simulink model "model5"  (R2022a)
settings: Solver=FixedStepAuto  StartTime=0.0  StopTime=20  FixedStep=1e-4  RelTol=1e-3
PreLoadFcn:
  | m = 3.600;     % kg
  | k = 400;    % N/m
  | b = 10;      % Ns/m
  | x0=1; %m
model workspace (MAT data in the model file):
  b1 = 10
  b2 = 10
  downSpringHeight = 10
  g = 9.81
  groundHeight = 100
  k1 = 400
  k2 = 400
  m1 = 3.6
  m1IniHeight = 10
  m2 = 3.6
  m3 = 3.6
  upSpringHeight = 10
settings Model: Creator=Tsing  LastModifiedBy=Tsing

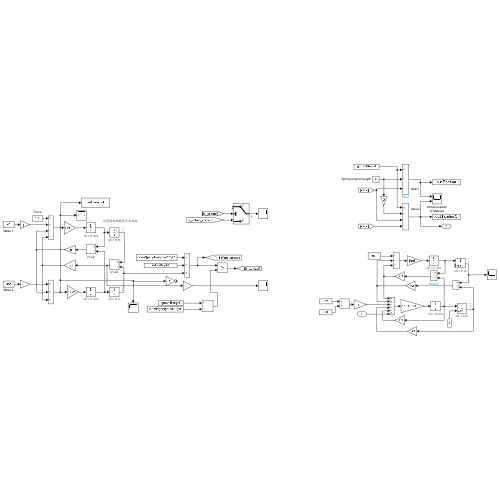
[thumbnail: Simulink's stored preview of the top-level diagram]
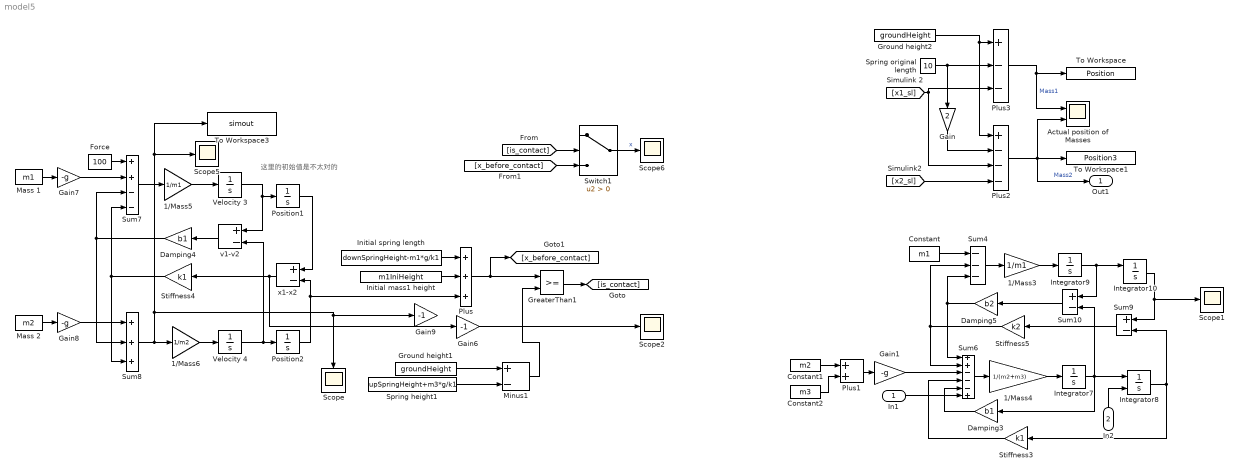
== system model5 ==
  note: 这里的初始值是不太对的
  In1 : Inport
  In2 : Inport  Port=2
  1/Mass3 : Gain  Gain=1/m1  SaturateOnIntegerOverflow=on  OutDataTypeStr=Inherit: Same as input  ParamDataTypeStr=Inherit: Same as input
  1/Mass4 : Gain  Gain=1/(m2+m3)  SaturateOnIntegerOverflow=on  OutDataTypeStr=Inherit: Same as input  ParamDataTypeStr=Inherit: Same as input
  1/Mass5 : Gain  Gain=1/m1  SaturateOnIntegerOverflow=on  OutDataTypeStr=Inherit: Same as input  ParamDataTypeStr=Inherit: Same as input
  1/Mass6 : Gain  Gain=1/m2  SaturateOnIntegerOverflow=on  OutDataTypeStr=Inherit: Same as input  ParamDataTypeStr=Inherit: Same as input
  Actual position of Masses : Scope  NumInputPorts=2
  Constant : Constant  Value=m1
  Constant1 : Constant  Value=m2
  Constant2 : Constant  Value=m3
  Damping3 : Gain  Gain=b1  SaturateOnIntegerOverflow=on  OutDataTypeStr=Inherit: Same as input  ParamDataTypeStr=Inherit: Same as input
  Damping4 : Gain  Gain=b1  SaturateOnIntegerOverflow=on  OutDataTypeStr=Inherit: Same as input  ParamDataTypeStr=Inherit: Same as input
  Damping5 : Gain  Gain=b2  SaturateOnIntegerOverflow=on  OutDataTypeStr=Inherit: Same as input  ParamDataTypeStr=Inherit: Same as input
  Force : Constant  Value=100
  Gain : Gain  Gain=2
  Gain1 : Gain  Gain=-g
  Gain6 : Gain  Gain=-1
  Gain7 : Gain  Gain=-g
  Gain8 : Gain  Gain=-g
  Gain9 : Gain  Gain=-1
  GreaterThan1 : RelationalOperator  OutDataTypeStr=boolean  RndMeth=Simplest  InputSameDT=off
  Ground height1 : Constant  Value=groundHeight
  Ground height2 : Constant  Value=groundHeight
  Initial mass1 height : Constant  Value=m1IniHeight
  Initial spring length : Constant  Value=downSpringHeight-m1*g/k1
  Integrator10 : Integrator  InitialConditionSource=external
      settings: AttributesFormatString=x0 = %<InitialCondition> m
  Integrator7 : Integrator
      settings: AttributesFormatString=v0 = %<InitialCondition> m/s
  Integrator8 : Integrator  InitialConditionSource=external
      settings: AttributesFormatString=x0 = %<InitialCondition> m
  Integrator9 : Integrator
      settings: AttributesFormatString=v0 = %<InitialCondition> m/s
  Mass 1 : Constant  Value=m1
  Mass 2 : Constant  Value=m2
  Minus1 : Sum  Inputs=+-
  Plus : Sum  Inputs=+++
  Plus1 : Sum
  Plus2 : Sum  Inputs=+---
  Plus3 : Sum  Inputs=+--
  Position1 : Integrator
      settings: AttributesFormatString=x0 = %<InitialCondition> m
  Position2 : Integrator
      settings: AttributesFormatString=x0 = %<InitialCondition> m
  Scope{,1..2,5..6} (5 alike) : Scope
  Spring height1 : Constant  Value=upSpringHeight+m3*g/k1
  Spring original length : Constant  Value=10
  Stiffness3 : Gain  Gain=k1  SaturateOnIntegerOverflow=on  OutDataTypeStr=Inherit: Same as input  ParamDataTypeStr=Inherit: Same as input
  Stiffness4 : Gain  Gain=k1  SaturateOnIntegerOverflow=on  OutDataTypeStr=Inherit: Same as input  ParamDataTypeStr=Inherit: Same as input
  Stiffness5 : Gain  Gain=k2  SaturateOnIntegerOverflow=on  OutDataTypeStr=Inherit: Same as input  ParamDataTypeStr=Inherit: Same as input
  Sum10 : Sum  Inputs=+-  InputSameDT=on  SaturateOnIntegerOverflow=on  OutDataTypeStr=Inherit: Same as first input
  Sum4 : Sum  Inputs=---  InputSameDT=on  SaturateOnIntegerOverflow=on  OutDataTypeStr=Inherit: Same as first input
  Sum6 : Sum  Inputs=++---+  InputSameDT=on  SaturateOnIntegerOverflow=on  OutDataTypeStr=Inherit: Same as first input
  Sum7 : Sum  Inputs=++--  InputSameDT=on  SaturateOnIntegerOverflow=on  OutDataTypeStr=Inherit: Same as first input
  Sum8 : Sum  Inputs=+++  InputSameDT=on  SaturateOnIntegerOverflow=on  OutDataTypeStr=Inherit: Same as first input
  Sum9 : Sum  Inputs=+-  InputSameDT=on  SaturateOnIntegerOverflow=on  OutDataTypeStr=Inherit: Same as first input
  Switch1 : Switch  Criteria=u2 > Threshold  SaturateOnIntegerOverflow=off  InputSameDT=off
  To Workspace : ToWorkspace  VariableName=Position  SaveFormat=Timeseries  SampleTime=-1
  To Workspace1 : ToWorkspace  VariableName=Position3  SaveFormat=Timeseries  SampleTime=-1
  To Workspace3 : ToWorkspace  VariableName=simout  SaveFormat=Timeseries  SampleTime=-1
  Velocity 3 : Integrator
      settings: AttributesFormatString=v0 = %<InitialCondition> m/s
  Velocity 4 : Integrator
      settings: AttributesFormatString=v0 = %<InitialCondition> m/s
  v1-v2 : Sum  Inputs=+-
  x1-x2 : Sum  Inputs=+-
  Out1 : Outport
  wires:
  Gain8/1 -> Sum8/1
  Mass 2/1 -> Gain8/1
  Sum8/1 -> To Workspace3/1, Scope5/1, Gain9/1, Scope/1, 1/Mass6/1
  Stiffness4/1 -> Sum7/4, Sum8/3
  Velocity 3/1 -> Position1/1, v1-v2/1
  Damping4/1 -> Sum7/3, Sum8/2
  Force/1 -> Sum7/1
  v1-v2/1 -> Damping4/1
  1/Mass5/1 -> Velocity 3/1
  Sum7/1 -> 1/Mass5/1
  Velocity 4/1 -> Position2/1, v1-v2/2
  Position1/1 -> x1-x2/1
  1/Mass6/1 -> Velocity 4/1
  Mass 1/1 -> Gain7/1
  Gain7/1 -> Sum7/2
  Position2/1 -> Plus/3, x1-x2/2
  x1-x2/1 -> Gain6/1, Stiffness4/1
  Spring height1/1 -> Minus1/2
  Ground height1/1 -> Minus1/1
  Plus/1 -> [x_before_contact], GreaterThan1/1
  Initial spring length/1 -> Plus/1
  Minus1/1 -> GreaterThan1/2
  GreaterThan1/1 -> [is_contact]
  Initial mass1 height/1 -> Plus/2
  Integrator10/1 -> Scope1/1, Sum9/1
  Stiffness3/1 -> Sum6/4
  Plus3/1 -> To Workspace/1, Actual position of Masses/1  "Mass1"
  Ground height2/1 -> Plus2/1, Plus3/1
  [x1_sl] -> Plus2/3, Plus3/3
  Sum9/1 -> Stiffness5/1
  1/Mass4/1 -> Integrator7/1
  In2/1 -> Integrator8/2
  Integrator7/1 -> Sum10/2, Integrator8/1, Damping3/1
  Gain/1 -> Plus2/2
  Spring original length/1 -> Gain/1, Plus3/2
  [x2_sl] -> Plus2/4
  Stiffness5/1 -> Sum6/2, Sum4/2
  Damping3/1 -> Sum6/5
  Integrator9/1 -> Integrator10/1, Sum10/1
  In1/1 -> Sum6/6
  Constant/1 -> Sum4/1
  Integrator8/1 -> Sum9/2, Stiffness3/1
  Plus2/1 -> Out1/1, To Workspace1/1, Actual position of Masses/2  "Mass2"
  Sum6/1 -> 1/Mass4/1
  Damping5/1 -> Sum4/3, Sum6/1
  Sum10/1 -> Damping5/1
  1/Mass3/1 -> Integrator9/1
  Sum4/1 -> 1/Mass3/1
  [is_contact] -> Switch1/2
  Switch1/1 -> Scope6/1  "x"
  [x_before_contact] -> Switch1/3
  Constant1/1 -> Plus1/1
  Constant2/1 -> Plus1/2
  Plus1/1 -> Gain1/1
  Gain1/1 -> Sum6/3
  Gain6/1 -> Scope2/1
